simulink model "RE4"  (R2020a)
settings: Solver=VariableStepAuto  StartTime=0.0  StopTime=10  RelTol=1e-3
undefined symbols (not defined in the file): Acid, Lead, sigbuilder_block
libraries: powerlib x20, re_lib x2, electricdrivelib x1
settings Model: Creator=deepv  LastModifiedBy=mitch

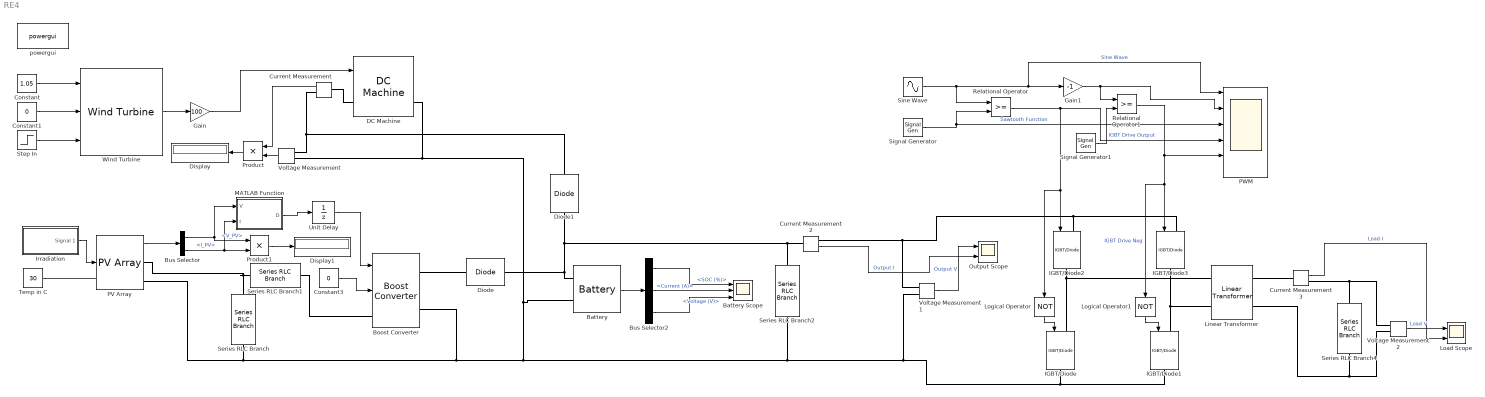
== system RE4 ==
  Battery : electricdrivelib/Extra Sources/Battery  BatType=Lead-Acid  ShowTempParam=off  ThermalPreset=no  ShowAgeParam=off  NomV=48  NomQ=2490  SOC=60  Batt_Tr=30  PresetModel=on  MaxQ=2593.75  MinV=36  FullV=52.2632  Dis_rate=498  R=0.00019277  Normal_OP=772.5917  expZone="[48.8684          8.3]"  current=[6.5 13 32.5]  Units=Time  Tci=20  NomT=20  T2=-30  MaxQ2=4.8  FullV2=7.1  Normal_OP2=5.655  expZone2="[6.58           1]"  Rca=0.6  ti=2000  Dp=0  Neq0=0  Tsim=1e6  Ta1=25  Qeol=5.4*0.9  Reol=0.013333*1.2  Char_age=[2.3478, 3]  Dis_age=[2.3478, 10]  N1=1500  N2=10500  N3=1000  N4=1400  Ta2=45  N5=950
  Battery Scope : Scope  NumInputPorts=3
  Boost Converter : powerlib/Power Electronics/Boost Converter  ModelType=Average model (D-controlled)  Ron=1e-3  Rs=1e6  Cs=inf  Vforward=[0,0]  Ron_Diode=1e-3  Rs_Diode=1e6  Cs_Diode=inf  Vf_Diode=1e-3  Rs_CurrentSource=inf
      settings: SourceProductBaseCode=PS
  Bus Selector : BusSelector  OutputSignals=V_PV,I_PV
  Bus Selector2 : BusSelector  OutputSignals=SOC (%),Current (A),Voltage (V)
  Constant : Constant  Value=1.05
  Constant1 : Constant  Value=0
  Constant3 : Constant  Value=0
  Current Measurement : powerlib/Measurements/Current Measurement  PhasorSimulation=off  OutputType=Complex  PSBequivalent=0
  Current Measurement2 : powerlib/Measurements/Current Measurement  PhasorSimulation=off  OutputType=Complex  PSBequivalent=0
  Current Measurement3 : powerlib/Measurements/Current Measurement  PhasorSimulation=off  OutputType=Complex  PSBequivalent=0
  DC Machine : powerlib/Machines/DC Machine  PresetModel=No  MechanicalLoad=Torque TL  FieldType=Permanent magnet  ShowDetailedParameters=on  MeasurementBus=off  RLa="[ 0.6  0.012]"  RLf="[ 240  120]"  Laf=1.8  MachineConstant=Torque constant (N.m/A)  Ke=1.8  Kt=1.8  J=1  Bm=0  Tf=0  w0=0  Ifinit=1  TsPowergui=0  TsBlock=-1
  Diode : powerlib/Power Electronics/Diode  Ron=0.001  Lon=0  Vf=0.8  IC=0  UseSnubber=0  Rs=500  Cs=250e-9  Measurements=off
  Diode1 : powerlib/Power Electronics/Diode  Ron=0.001  Lon=0  Vf=0.8  IC=0  UseSnubber=0  Rs=500  Cs=250e-9  Measurements=off
  Display : Display
  Display1 : Display
  Gain : Gain  Gain=100
  Gain1 : Gain  Gain=-1
  IGBT/Diode{,1..3} (4 alike) : powerlib/Power Electronics/IGBT//Diode  Ron=1e-3  Rs=1e5  Cs=inf  Measurements=off
  Irradiation : Subsystem  Tag=STV Subsys  LoadFcn=sigbuilder_block('load');  StartFcn=sigbuilder_block('start');  StopFcn=sigbuilder_block('stop');  ClipboardFcn=sigbuilder_block('clipboard');  mask(Sigbuilder block){tuvar=[0:10]}
      mask help: Simulink:masks:SigbuilderBlock_MD
      mask init:
      | if ~strcmp(get_param(bdroot(gcbh),'SimulationStatus'),'stopped') tuvar = sigbuilder_block('maskInit'); end
      settings: CopyFcn=sigbuilder_block('copy');  DeleteFcn=sigbuilder_block('delete');  ModelCloseFcn=sigbuilder_block('modelClose');  PreSaveFcn=sigbuilder_block('preSave');  PauseFcn=sigbuilder_block('pause');  ContinueFcn=sigbuilder_block('continue');  NameChangeFcn=sigbuilder_block('namechange');  OpenFcn=sigbuilder_block('open',[133.234 117.757 550.43 399.701 ]);  CloseFcn=sigbuilder_block('close');
      mask Display: plot(0, 0, 100, 100,[2, 2, 32, 32, 2], [68, 8, 8, 68, 68],[32, 2], [38, 38], [32, 19, 2],[53, 60, 44], [32, 17, 17, 2],[16, 16, 31, 31]);txt = getActiveGroup(gcbh);text(2, 100, txt,'verticalAlignment', 'top');
  Linear Transformer : powerlib/Elements/Linear Transformer  UNITS=SI  NominalPower=[ 250e6 60 ]  winding1=[7.35e+05 4.3218 0.45856]  winding2=[3.15e+05 0.7938 0.084225]  ThreeWindings=off  winding3=[3.15e+05 0.7938 0.084225]  RmLm=[1.0805e+06 2866]  Measurements=None  DataType=on
  Load Scope : Scope  NumInputPorts=2
  Logical Operator : Logic  Operator=NOT  AllPortsSameDT=off  OutDataTypeStr=boolean
  Logical Operator1 : Logic  Operator=NOT  AllPortsSameDT=off  OutDataTypeStr=boolean
  MATLAB Function : MATLAB Function  TreatAsAtomicUnit=on
  Output Scope : Scope  NumInputPorts=2
  PV Array : re_lib/Solar/PV Array  Npar=40  Nser=2  PlotType=array @ 1000 W/m2 & specified temperatures  S_vec="[ 1000  500  100 ]"  Temp_C_vec="[ 30  ]"  ModuleName=User-defined  PlotWhenSelected=off  Pm=189.888  Ncell=72  Voc=45  Isc=5.56  Vm=36.8  Im=5.16  beta_Voc_pc=-0.33  alpha_Isc_pc=0.065  beta_Voc=-0.1485  alpha_Isc=0.003614  IL=5.5761  I0=6.3584e-11  nI=0.96666  Rsh=257.6724  Rs=0.54375  RobustModel=on  RobustCellTemperature=25  BAL=on  Tc=1e-6  Tfilter=5e-5
  PWM : Scope  NumInputPorts=6
  Product : Product
  Product1 : Product
  Relational Operator : RelationalOperator  OutDataTypeStr=boolean  RndMeth=Simplest
  Relational Operator1 : RelationalOperator  OutDataTypeStr=boolean  RndMeth=Simplest
  Series RLC Branch : powerlib/Elements/Series RLC Branch  LConnTagsString=__new0  RConnTagsString=__new0  BranchType=C  Resistance=1  Inductance=1e-3  SetiL0=off  InitialCurrent=0  Capacitance=1e-6  Setx0=off  InitialVoltage=0  Measurements=None
  Series RLC Branch1 : powerlib/Elements/Series RLC Branch  LConnTagsString=__new0  RConnTagsString=__new0  BranchType=L  Resistance=1  Inductance=1e-3  SetiL0=off  InitialCurrent=0  Capacitance=1e-6  Setx0=off  InitialVoltage=0  Measurements=None
  Series RLC Branch2 : powerlib/Elements/Series RLC Branch  LConnTagsString=__new0  RConnTagsString=__new0  BranchType=C  Resistance=1  Inductance=1e-3  SetiL0=off  InitialCurrent=0  Capacitance=1e-6  Setx0=off  InitialVoltage=0  Measurements=None
  Series RLC Branch4 : powerlib/Elements/Series RLC Branch  LConnTagsString=__new0  RConnTagsString=__new0  BranchType=RL  Resistance=5.44  Inductance=0.00406  SetiL0=off  InitialCurrent=0  Capacitance=1e-6  Setx0=off  InitialVoltage=0  Measurements=None
  Signal Generator : SignalGenerator  WaveForm=sawtooth  Amplitude=311  Frequency=15000
  Signal Generator1 : SignalGenerator  WaveForm=sawtooth  Amplitude=311  Frequency=15000
  Sine Wave : Sin  Amplitude=311*sqrt(2)  Frequency=50*2*pi  SampleTime=0
  Step In : Step  Time=5  Before=11  After=12  SampleTime=0
  Temp in C : Constant  Value=30
  "Unit Delay " : UnitDelay  SampleTime=-1  HasFrameUpgradeWarning=on
  Voltage Measurement : powerlib/Measurements/Voltage Measurement  PhasorSimulation=off  OutputType=Complex  PSBequivalent=0
  Voltage Measurement1 : powerlib/Measurements/Voltage Measurement  PhasorSimulation=off  OutputType=Complex  PSBequivalent=0
  Voltage Measurement2 : powerlib/Measurements/Voltage Measurement  PhasorSimulation=off  OutputType=Complex  PSBequivalent=0
  Wind Turbine : re_lib/Wind Generation/Wind Turbine  Pnom=10000  Pelec_base=10000/0.9  wind_base=12  P_wind_base=0.73  speed_nom=1.2  pitch_angle=0  c1_c6="[0.51763          116          0.4            5           21     0.006795]"  cp_nom=0.48  lambda_nom=8.1
      settings: SourceProductBaseCode=PS
  powergui : powerlib/powergui  Priority=1  SimulationMode=Discrete  SampleTime=50e-6  frequency=60  Iterations=50  frequencyindice=0  Pbase=100e6  ErrMax=1e-4  UnitsV=kV  UnitsW=MW  buscounter=0  FunctionMessages=off  echomessages=off  EnableUseOfTLC=off  CurrentSourceSwitches=off  DisableSnubberDevices=off  DisableRonSwitches=off  DisableVfSwitches=off  DisplayEquations=off  AutomaticDiscreteSolvers=off  SolverType=Tustin/Backward Euler (TBE)  Interpol=off  ExternalGateDelay=off  methode=off  Ts=100  x0status=blocks  SPID=on  SwTol=0  HookPort=off  NonlinearTolerance=1e-4  nMaxIteration=100  ContinueOnMaxIteration=off  RestoreLinks=warning  ResistiveCurrentMeasurement=off  Frange=[0:2:500]  Ylog=off  Xlog=on  ShowGrid=off  save=off  variable=ZData  structure=0  ZoomFFT=off  StartTime=0.0  cycles=1  DisplayStyle=1  fundamental=60  FreqAxis=off  MaxFrequency=1000  frequencyindicesteady=1  RmsSteady=1  display=off
  wires:
  Constant1/1 -> Wind Turbine/2
  Constant/1 -> Wind Turbine/1
  Step In/1 -> Wind Turbine/3
  Irradiation/1(Signal 1) -> PV Array/1
  Temp in C/1 -> ?
  Wind Turbine/1 -> Gain/1
  Gain/1 -> DC Machine/1
  Voltage Measurement/1 -> Product/2
  Current Measurement/1 -> Product/1
  Product/1 -> Display/1
  Bus Selector/2 -> MATLAB Function/2(I), Product1/2  "<I_PV>"
  Bus Selector/1 -> MATLAB Function/1(V), Product1/1  "<V_PV>"
  PV Array/1 -> Bus Selector/1
  Product1/1 -> Display1/1
  MATLAB Function/1(D) -> "Unit Delay "/1
  "Unit Delay "/1 -> Boost Converter/1
  Constant3/1 -> Boost Converter/2
  Bus Selector2/3 -> Battery Scope/3  "<Voltage (V)>"
  Bus Selector2/2 -> Battery Scope/2  "<Current (A)>"
  Bus Selector2/1 -> Battery Scope/1  "<SOC (%)>"
  Battery/1 -> Bus Selector2/1
  Current Measurement2/1 -> Output Scope/2  "Output I"
  Voltage Measurement1/1 -> Output Scope/1  "Output V"
  Signal Generator/1 -> PWM/3, Relational Operator/2  "Sawtooth Function"
  Sine Wave/1 -> PWM/1, Gain1/1, Relational Operator/1  "Sine Wave"
  Signal Generator1/1 -> Relational Operator1/2
  Gain1/1 -> PWM/2, Relational Operator1/1
  Relational Operator/1 -> PWM/4, IGBT/Diode2/1, Logical Operator/1  "IGBT Drive Output"
  Relational Operator1/1 -> PWM/5, IGBT/Diode3/1, Logical Operator1/1  "IGBT Drive Neg"
  Logical Operator/1 -> IGBT/Diode/1
  Logical Operator1/1 -> IGBT/Diode1/1
  Voltage Measurement2/1 -> Load Scope/1  "Load V"
  Current Measurement3/1 -> Load Scope/2  "Load I"
  connections:
  Current Measurement/LConn1 -- DC Machine/LConn1
  Current Measurement/RConn1 -- Diode1/LConn1 -- Voltage Measurement/LConn1
  Voltage Measurement1/LConn2 -- Battery/LConn2 -- Voltage Measurement/LConn2 -- DC Machine/RConn1 -- Boost Converter/RConn2 -- Series RLC Branch/RConn1 -- PV Array/RConn2 -- Series RLC Branch2/RConn1 -- IGBT/Diode1/RConn1 -- IGBT/Diode/RConn1
  Diode/LConn1 -- Boost Converter/RConn1
  Battery/LConn1 -- Series RLC Branch2/LConn1 -- Current Measurement2/LConn1 -- Diode1/RConn1 -- Diode/RConn1
  PV Array/RConn1 -- Series RLC Branch1/LConn1 -- Series RLC Branch/LConn1
  Series RLC Branch1/RConn1 -- Boost Converter/LConn1
  Current Measurement2/RConn1 -- Voltage Measurement1/LConn1 -- IGBT/Diode3/LConn1 -- IGBT/Diode2/LConn1
  IGBT/Diode1/LConn1 -- IGBT/Diode3/RConn1 -- Linear Transformer/LConn2
  IGBT/Diode2/RConn1 -- IGBT/Diode/LConn1 -- Linear Transformer/LConn1
  Linear Transformer/RConn1 -- Current Measurement3/LConn1
  Current Measurement3/RConn1 -- Series RLC Branch4/LConn1 -- Voltage Measurement2/LConn1
  Voltage Measurement2/LConn2 -- Series RLC Branch4/RConn1 -- Linear Transformer/RConn2

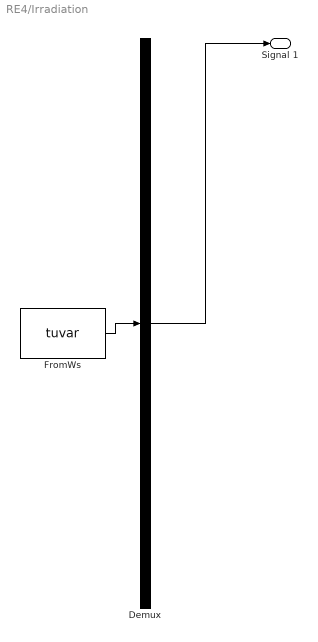
== system RE4/Irradiation ==
  Demux : Demux  Tag=STV Demux  Outputs=1
      settings: DisplayOption=none
  FromWs : FromWorkspace  Tag=STV FromWs  VariableName=tuvar
      SigBuilderData=|
      | common.afterFinalStr = 'Extrapolate'
      | common.sampleTime = 0
      | dataSet.timeRange = [0 20]
      | dataSet.name = 'Group 1'
      | sbobj.Groups.Name = 'Group 1'
      | sbobj.Groups.Signals.Name = 'Signal 1'
      | sbobj.Groups.Signals.XData = [0 3 4 6 20]
      | sbobj.Groups.Signals.YData = [400 400 1000 1000 1000]
      | sbobj.Groups.TimeRange = [0 20]
  Signal 1 : Outport  Tag=STV Outport
  wires:
  Demux/1 -> Signal 1/1
  FromWs/1 -> Demux/1

== matlab function RE4/MATLAB Function ==
  data: V input; D output; I input
function D = fcn(V,I)

dD=0.00001;
Dmin=0.2;
Dmax=0.8;
Vinital=0;
Iinitial=0;
Dinitial=0.41;

persistent Vold Iold Dold;

isempty(V)
Vold=Vinital;
Iold=Iinitial;
Dold=Dinitial;

dI=I-Iold;
dV=V-Vold;

if V * dI + I * dV == 0
    D = Dold
else
    if V * dI + I * dV > 0
        D = Dold + dD
    else
        D = Dold - dD
    end
end

if D >= Dmax||D <= Dmin
    D = Dold;
end

Vold=V;
Iold=I;
Dold=D;
